simulink model "MPC_Extended_Plant_Simulink"  (R2023b)
settings: Solver=ode4  StartTime=0.0  StopTime=20  FixedStep=1e-3  RelTol=1e-3
values from neighbouring files (symbols this model uses):
  controller_choice = input('Select MPC controller order (1, 2, or 3): ')    [MPC_Extended_Plant.m]    (also in P1.mat = 1; P2.mat = 2; P3.mat = 3)
  init =     [P1.mat]    (also in P2.mat; P3.mat)
  input =     [P1.mat]    (also in P2.mat; P3.mat)
  Np = 40    [MPC_Extended_Plant.m]    (also in P1.mat = 5; P2.mat = 5; P3.mat = 5)
  par =     [P1.mat]    (also in P2.mat; P3.mat)
  Ts = 0.01    [MPC_Extended_Plant.m]    (also in P1.mat; P2.mat; P3.mat)
  V_ref = 16.6666666667    [P1.mat]    (also in P2.mat; P3.mat; veh_parameters.m)
undefined symbols (not defined in the file or in its folder): data
libraries: simulink x12
(part 1 of 2)
settings Model: Creator=bshyrokau  LastModifiedBy=india
settings SolverCC: AlgebraicLoopSolver=TrustRegion
settings DataIOCC: SaveOutput=off  SignalLogging=off  DSMLogging=off  SaveTime=off  ReturnWorkspaceOutputs=off
settings OptimizationCC: ReuseModelBlockBuffer=off  LifeSpan=inf
settings DebuggingCC: UnconnectedInputMsg=warning  UnconnectedOutputMsg=warning  UnconnectedLineMsg=warning  AllowSymbolicDim=off  SFUnexpectedBacktrackingDiag=warning  SFNoUnconditionalDefaultTransitionDiag=warning  SFExecutionAtInitializationDiag=none  ArithmeticOperatorsInVariantConditions=warning
settings ModelReferenceCC: EnableRefExpFcnMdlSchedulingChecks=on  PropagateSignalLabelsOutOfModel=off
settings SFSimCC: SimUseLocalCustomCode=off  CustomCodeUndefinedFunction=UseInterfaceOnly
settings RTWCC: RTWUseLocalCustomCode=off  DLArmComputeVersion=19.05
settings CodeAppCC: StateflowObjectComments=on
settings GRTTargetCC: TargetLangStandard=C89/C90 (ANSI)
settings ConfigComp: CovMetricSettings=dw  CovSaveCumulativeToWorkspaceVar=on  CovSaveSingleToWorkspaceVar=on  CovExternalEMLEnable=off
settings SimscapeCC: SimscapeNormalizeSystem=off
settings ConfigurationSet: Description=SimMechanics 2G

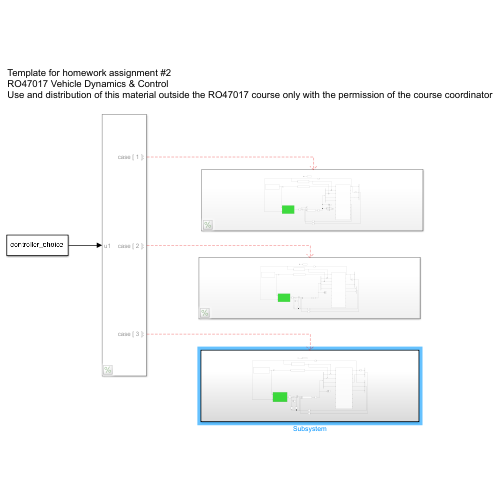
[thumbnail: Simulink's stored preview of the top-level diagram]
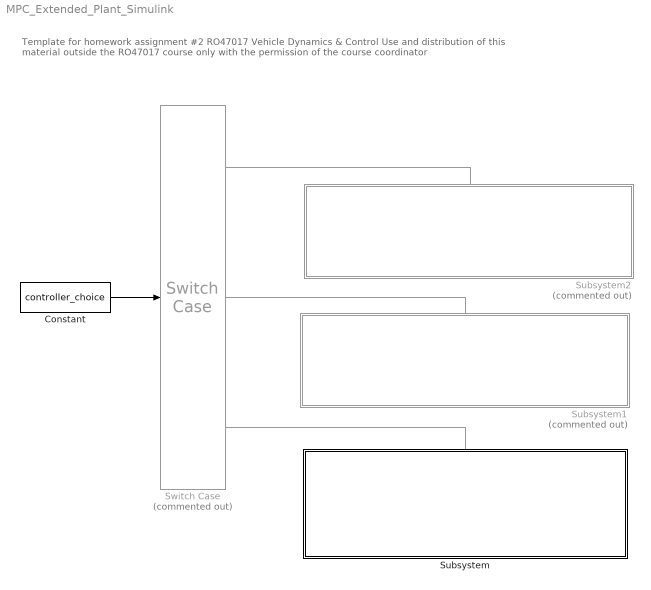
== system MPC_Extended_Plant_Simulink ==
  note: Template for homework assignment #2
      | RO47017 Vehicle Dynamics & Control
      | Use and distribution of this material outside the RO47017 course only with the permission of the course coordinator
  Constant : Constant  Value=controller_choice
  Subsystem : Subsystem
  Subsystem1 : Subsystem  Commented=on
  Subsystem2 : Subsystem  Commented=on
  Switch Case : SwitchCase  Commented=on  CaseConditions={1 2 3}  ShowDefaultCase=off
  wires:
  Switch Case/2 -> ?
  Switch Case/3 -> ?
  Constant/1 -> Switch Case/1
  Switch Case/1 -> ?

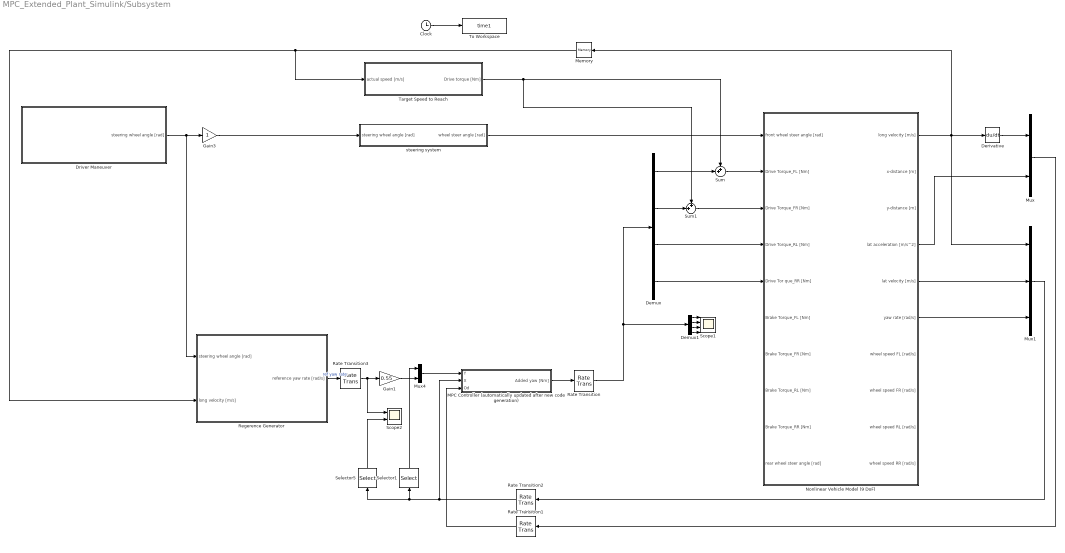
== system MPC_Extended_Plant_Simulink/Subsystem ==
  Clock : Clock
  Demux : Demux
  Demux1 : Demux
  Derivative : Derivative
  Driver Maneuver : Subsystem
  Gain1 : Gain  Gain=0.55
  Gain3 : Gain
  MPC Controller (automatically updated after new code generation) : Subsystem
  Memory : Memory  InitialCondition=V_ref
  Mux : Mux  Inputs=2
  Mux1 : Mux  Inputs=3
  Mux4 : Mux  Inputs=2
  Nonlinear Vehicle Model (9 DoF) : Subsystem
      mask help: Simulink:masks:GenSFuncDesc_MD
      mask Help: eval('feval(''rtwprivate'',''rtwhelpview'',''rtw_sfcn_block'')');
  Rate Transition : RateTransition
  Rate Transition1 : RateTransition  InitialCondition=[0 0]  OutPortSampleTime=Ts
  Rate Transition2 : RateTransition  OutPortSampleTime=Ts
  Rate Transition3 : RateTransition  OutPortSampleTime=Ts
  Regerence Generator : Subsystem
  Scope1 : Scope  NumInputPorts=4
  Scope2 : Scope  NumInputPorts=2
  Selector1 : Selector  InputPortWidth=3  IndexOptions=Index vector (dialog)  Indices=[1 2]  OutputSizes=1
  Selector5 : Selector  InputPortWidth=3  IndexOptions=Index vector (dialog)  Indices=3  OutputSizes=1
  Sum : Sum  Inputs=++|
  Sum1 : Sum  Inputs=++|
  Target Speed to Reach : Subsystem
  To Workspace : ToWorkspace  VariableName=time1  SampleTime=-1
  steering system : Subsystem
  wires:
  Gain1/1 -> Mux4/2
  Selector1/1 -> Mux4/1
  Selector5/1 -> Scope2/2
  Regerence Generator/1(reference yaw rate [rad/s]) -> Rate Transition3/1  "ref yaw rate"
  Target Speed to Reach/1(Drive torque [Nm]) -> Sum/1, Sum1/1
  Demux1/4 -> Scope1/4
  MPC Controller (automatically updated after new code generation)/1(Added yaw [Nm]) -> Rate Transition/1
  Demux/1 -> Sum/2
  Gain3/1 -> steering system/1(steering wheel angle [rad])
  Memory/1 -> Target Speed to Reach/1(actual speed [m/s]), Regerence Generator/2(long velocity [m/s])
  Nonlinear Vehicle Model (9 DoF)/1(long velocity [m/s]) -> Derivative/1, Memory/1, Mux1/1
  Sum/1 -> Nonlinear Vehicle Model (9 DoF)/2(Drive Torque_FL [Nm])
  steering system/1(wheel steer angle [rad]) -> Nonlinear Vehicle Model (9 DoF)/1(front wheel steer angle [rad])
  Rate Transition/1 -> Demux1/1, Demux/1
  Demux1/1 -> Scope1/1
  Demux/3 -> Nonlinear Vehicle Model (9 DoF)/4(Drive Torque_RL [Nm])
  Demux/4 -> Nonlinear Vehicle Model (9 DoF)/5(Drive Tor	que_RR [Nm])
  Demux1/2 -> Scope1/2
  Driver Maneuver/1(steering wheel angle [rad]) -> Gain3/1, Regerence Generator/1(steering wheel angle [rad])
  Mux4/1 -> MPC Controller (automatically updated after new code generation)/1(Y)
  Clock/1 -> To Workspace/1
  Sum1/1 -> Nonlinear Vehicle Model (9 DoF)/3(Drive Torque_FR [Nm])
  Rate Transition2/1 -> Selector5/1, Selector1/1, MPC Controller (automatically updated after new code generation)/2(X)
  Mux1/1 -> Rate Transition2/1
  Demux/2 -> Sum1/2
  Demux1/3 -> Scope1/3
  Rate Transition3/1 -> Scope2/1, Gain1/1
  Nonlinear Vehicle Model (9 DoF)/6(yaw rate [rad/s]) -> Mux1/3
  Nonlinear Vehicle Model (9 DoF)/5(lat velocity [m/s]) -> Mux1/2
  Derivative/1 -> Mux/1
  Nonlinear Vehicle Model (9 DoF)/4(lat acceleration [m/s^2]) -> Mux/2
  Mux/1 -> Rate Transition1/1
  Rate Transition1/1 -> MPC Controller (automatically updated after new code generation)/3(Od)

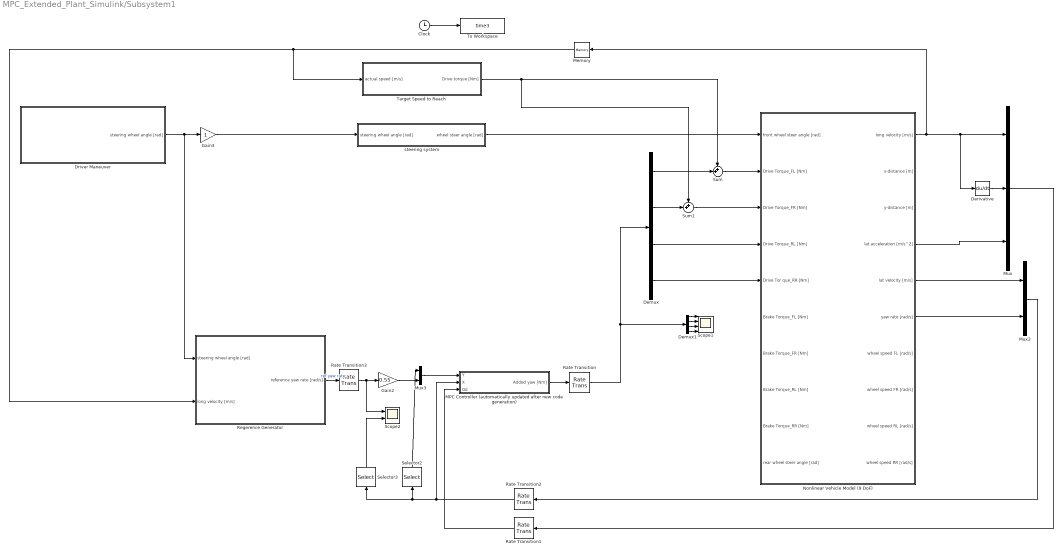
== system MPC_Extended_Plant_Simulink/Subsystem1 ==
  Clock : Clock
  Demux : Demux
  Demux1 : Demux
  Derivative : Derivative
  Driver Maneuver : Subsystem
  Gain2 : Gain  Gain=0.55
  Gain3 : Gain
  MPC Controller (automatically updated after new code generation) : Subsystem
  Memory : Memory  InitialCondition=V_ref
  Mux : Mux  Inputs=3
  Mux2 : Mux  Inputs=2
  Mux3 : Mux  Inputs=2
  Nonlinear Vehicle Model (9 DoF) : Subsystem
      mask help: Simulink:masks:GenSFuncDesc_MD
      mask Help: eval('feval(''rtwprivate'',''rtwhelpview'',''rtw_sfcn_block'')');
  Rate Transition : RateTransition
  Rate Transition1 : RateTransition  InitialCondition=[V_ref 0 0]  OutPortSampleTime=Ts
  Rate Transition2 : RateTransition  OutPortSampleTime=Ts
  Rate Transition3 : RateTransition  OutPortSampleTime=Ts
  Regerence Generator : Subsystem
  Scope1 : Scope  NumInputPorts=4
  Scope2 : Scope  NumInputPorts=2
  Selector2 : Selector  InputPortWidth=2  IndexOptions=Index vector (dialog)  Indices=1  OutputSizes=1
  Selector3 : Selector  InputPortWidth=2  IndexOptions=Index vector (dialog)  Indices=2  OutputSizes=1
  Sum : Sum  Inputs=++|
  Sum1 : Sum  Inputs=++|
  Target Speed to Reach : Subsystem
  To Workspace : ToWorkspace  VariableName=time3  SampleTime=-1
  steering system : Subsystem
  wires:
  Demux1/2 -> Scope1/2
  Demux1/1 -> Scope1/1
  Rate Transition/1 -> Demux1/1, Demux/1
  Demux/3 -> Nonlinear Vehicle Model (9 DoF)/4(Drive Torque_RL [Nm])
  Demux/4 -> Nonlinear Vehicle Model (9 DoF)/5(Drive Tor	que_RR [Nm])
  Sum/1 -> Nonlinear Vehicle Model (9 DoF)/2(Drive Torque_FL [Nm])
  steering system/1(wheel steer angle [rad]) -> Nonlinear Vehicle Model (9 DoF)/1(front wheel steer angle [rad])
  Nonlinear Vehicle Model (9 DoF)/1(long velocity [m/s]) -> Derivative/1, Mux/1, Memory/1
  Demux1/3 -> Scope1/3
  Memory/1 -> Target Speed to Reach/1(actual speed [m/s]), Regerence Generator/2(long velocity [m/s])
  Demux/1 -> Sum/2
  Gain3/1 -> steering system/1(steering wheel angle [rad])
  Demux1/4 -> Scope1/4
  MPC Controller (automatically updated after new code generation)/1(Added yaw [Nm]) -> Rate Transition/1
  Target Speed to Reach/1(Drive torque [Nm]) -> Sum/1, Sum1/1
  Regerence Generator/1(reference yaw rate [rad/s]) -> Rate Transition3/1  "ref yaw rate"
  Demux/2 -> Sum1/2
  Sum1/1 -> Nonlinear Vehicle Model (9 DoF)/3(Drive Torque_FR [Nm])
  Rate Transition3/1 -> Scope2/1, Gain2/1
  Clock/1 -> To Workspace/1
  Rate Transition2/1 -> Selector3/1, Selector2/1, MPC Controller (automatically updated after new code generation)/2(X)
  Driver Maneuver/1(steering wheel angle [rad]) -> Gain3/1, Regerence Generator/1(steering wheel angle [rad])
  Nonlinear Vehicle Model (9 DoF)/5(lat velocity [m/s]) -> Mux2/1
  Nonlinear Vehicle Model (9 DoF)/6(yaw rate [rad/s]) -> Mux2/2
  Mux2/1 -> Rate Transition2/1
  Mux3/1 -> MPC Controller (automatically updated after new code generation)/1(Y)
  Gain2/1 -> Mux3/2
  Selector2/1 -> Mux3/1
  Selector3/1 -> Scope2/2
  Nonlinear Vehicle Model (9 DoF)/4(lat acceleration [m/s^2]) -> Mux/3
  Derivative/1 -> Mux/2
  Mux/1 -> Rate Transition1/1
  Rate Transition1/1 -> MPC Controller (automatically updated after new code generation)/3(Od)

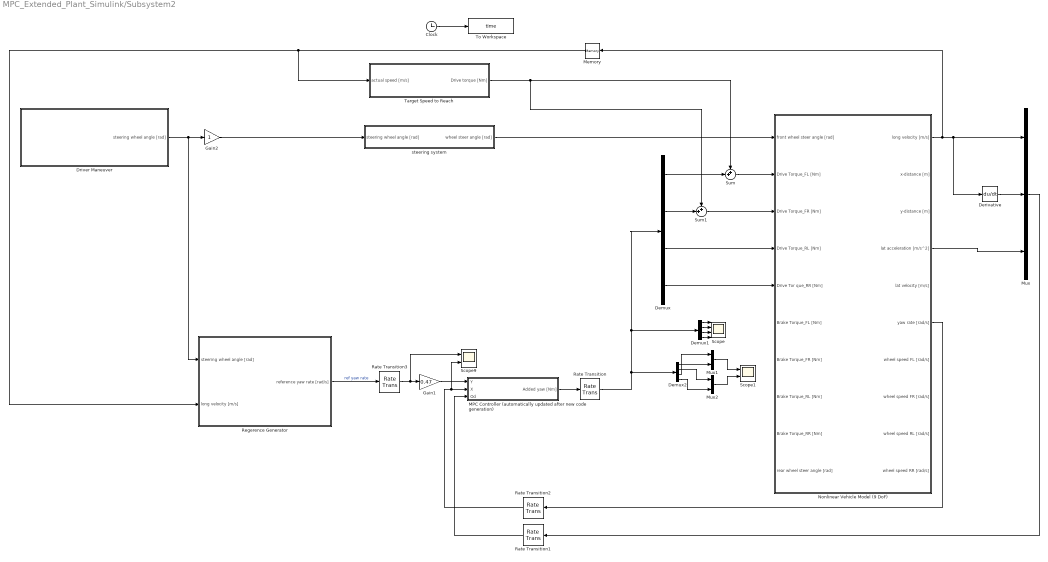
== system MPC_Extended_Plant_Simulink/Subsystem2 ==
  Clock : Clock
  Demux : Demux
  Demux1 : Demux
  Demux2 : Demux
  Derivative : Derivative
  Driver Maneuver : Subsystem
  Gain1 : Gain  Gain=0.47
  Gain2 : Gain
  MPC Controller (automatically updated after new code generation) : Subsystem
  Memory : Memory  InitialCondition=V_ref
  Mux : Mux  Inputs=3
  Mux1 : Mux  Inputs=2
  Mux2 : Mux  Inputs=2
  Nonlinear Vehicle Model (9 DoF) : Subsystem
      mask help: Simulink:masks:GenSFuncDesc_MD
      mask Help: eval('feval(''rtwprivate'',''rtwhelpview'',''rtw_sfcn_block'')');
  Rate Transition : RateTransition  InitialCondition=[0 0 0 0]
  Rate Transition1 : RateTransition  InitialCondition=[V_ref 0 0]  OutPortSampleTime=Ts
  Rate Transition2 : RateTransition  OutPortSampleTime=Ts
  Rate Transition3 : RateTransition  OutPortSampleTime=Ts
  Regerence Generator : Subsystem
  Scope : Scope  NumInputPorts=4
  Scope1 : Scope  NumInputPorts=2
  Scope9 : Scope  NumInputPorts=2
  Sum : Sum  Inputs=++|
  Sum1 : Sum  Inputs=++|
  Target Speed to Reach : Subsystem
  To Workspace : ToWorkspace  VariableName=time  SampleTime=-1
  steering system : Subsystem
  wires:
  MPC Controller (automatically updated after new code generation)/1(Added yaw [Nm]) -> Rate Transition/1
  Gain1/1 -> MPC Controller (automatically updated after new code generation)/1(Y)
  Rate Transition2/1 -> Scope9/2, MPC Controller (automatically updated after new code generation)/2(X)
  Rate Transition3/1 -> Gain1/1, Scope9/1
  Clock/1 -> To Workspace/1
  Regerence Generator/1(reference yaw rate [rad/s]) -> Rate Transition3/1  "ref yaw rate"
  Driver Maneuver/1(steering wheel angle [rad]) -> Gain2/1, Regerence Generator/1(steering wheel angle [rad])
  Gain2/1 -> steering system/1(steering wheel angle [rad])
  steering system/1(wheel steer angle [rad]) -> Nonlinear Vehicle Model (9 DoF)/1(front wheel steer angle [rad])
  Nonlinear Vehicle Model (9 DoF)/6(yaw rate [rad/s]) -> Rate Transition2/1
  Target Speed to Reach/1(Drive torque [Nm]) -> Sum/1, Sum1/1
  Memory/1 -> Target Speed to Reach/1(actual speed [m/s]), Regerence Generator/2(long velocity [m/s])
  Nonlinear Vehicle Model (9 DoF)/1(long velocity [m/s]) -> Memory/1, Derivative/1, Mux/1
  Demux/3 -> Nonlinear Vehicle Model (9 DoF)/4(Drive Torque_RL [Nm])
  Demux/4 -> Nonlinear Vehicle Model (9 DoF)/5(Drive Tor	que_RR [Nm])
  Demux/1 -> Sum/2
  Sum/1 -> Nonlinear Vehicle Model (9 DoF)/2(Drive Torque_FL [Nm])
  Sum1/1 -> Nonlinear Vehicle Model (9 DoF)/3(Drive Torque_FR [Nm])
  Demux/2 -> Sum1/2
  Rate Transition/1 -> Demux2/1, Demux1/1, Demux/1
  Demux1/1 -> Scope/1
  Demux1/2 -> Scope/2
  Demux1/3 -> Scope/3
  Demux1/4 -> Scope/4
  Nonlinear Vehicle Model (9 DoF)/4(lat acceleration [m/s^2]) -> Mux/3
  Derivative/1 -> Mux/2
  Rate Transition1/1 -> MPC Controller (automatically updated after new code generation)/3(Od)
  Mux/1 -> Rate Transition1/1
  Demux2/1 -> Mux1/1
  Demux2/3 -> Mux1/2
  Demux2/2 -> Mux2/1
  Demux2/4 -> Mux2/2
  Mux1/1 -> Scope1/1
  Mux2/1 -> Scope1/2

== system MPC_Extended_Plant_Simulink/Subsystem/Driver Maneuver ==
  Constant1 : Constant
  Lookup Table1 : Lookup  InputValues=[0:0.1:3*pi/2 3*pi/2+eps]*0.7  Table=sin([0:0.1:3*pi/2 3*pi/2+eps])  LookUpMeth=Interpolation-Use End Values  SaturateOnIntegerOverflow=off
  Lookup Table2 : Lookup  InputValues=[3*pi/2:0.1:2*pi 2*pi+eps]*0.7  Table=sin([3*pi/2:0.1:2*pi 2*pi+eps])  LookUpMeth=Interpolation-Use End Values  SaturateOnIntegerOverflow=off
  Ramp2 : simulink/Sources/Ramp  slope=1  start=10  InitialOutput=0
  Ramp6 : simulink/Sources/Ramp  slope=pi  start=10  InitialOutput=0
  Ramp7 : simulink/Sources/Ramp  slope=pi  start=10+0.5  InitialOutput=0
  Sine Wave : Sin  TimeSource=Use external signal  Amplitude=30/180*pi  Frequency=2*pi*0.2  SampleTime=0
  Subtract1 : Sum  Inputs=+++
  Terminator1 : Terminator
  amplitude : Gain  Gain=120
  deg2rad : Gain  Gain=pi / 180
  steering wheel angle [rad] : Outport  VectorParamsAs1DForOutWhenUnconnected=off
  wires:
  Ramp6/1 -> Lookup Table1/1
  Ramp7/1 -> Lookup Table2/1
  Lookup Table2/1 -> Subtract1/2
  Lookup Table1/1 -> Subtract1/1
  Constant1/1 -> Subtract1/3
  Subtract1/1 -> amplitude/1
  amplitude/1 -> deg2rad/1
  Ramp2/1 -> Sine Wave/1
  deg2rad/1 -> steering wheel angle [rad]/1
  Sine Wave/1 -> Terminator1/1

== system MPC_Extended_Plant_Simulink/Subsystem/MPC Controller (automatically updated after new code generation) ==
  Y : Inport
  X : Inport  Port=2
  Od : Inport  Port=3
  Bus Assignment : BusAssignment  AssignedSignals=data.x0,data.y,data.yN,data.W,data.WN,data.od
  Bus Creator : BusCreator  Inputs=4  OutDataTypeStr=Bus: ACADOinput
  Bus Selector : BusSelector  OutputSignals=data
  Bus Selector1 : BusSelector  OutputSignals=data.u
  Initial conditions : Constant  Value=[V_ref 0 0]
  Selector : Selector  InputPortWidth=Np*4  IndexOptions=Starting index (dialog)  Indices=1  OutputSizes=4
  Shift reference : MATLAB Function  TreatAsAtomicUnit=on
  Shift reference1 : MATLAB Function  TreatAsAtomicUnit=on
  Unit Delay : UnitDelay  InitialCondition=init  SampleTime=Ts  HasFrameUpgradeWarning=on
  acado_solver_sfun : S-Function  FunctionName=acado_solver_sfun  SFunctionDeploymentMode=off  EnableBusSupport=off  mask(Legacy Function){SFunctionSpec=acado_step(ACADOinput u1[1], ACADOoutput y1[1]), ShowSpec=on}
      mask prompts: ShowSpec "Display function specification"
      mask help:
      | This block allows you to call the legacy functions specified by the following Legacy Code Tool definition:
      | def.SFunctionName = 'acado_solver_sfun';
      | def.OutputFcnSpec = 'acado_step(ACADOinput u1[1], ACADOoutput y1[1])';
      | def.StartFcnSpec = 'acado_initialize( void )';
      | def.TerminateFcnSpec = 'acado_cleanup( void )';
      | def.HeaderFiles = {'acado_common.h', 'acado_solver_sfunction.h'};
      | def.SourceFiles = {'acado_solver.c', 'acado_integrator.c', 'acado_auxiliary_functions.c', 'acado_solver_sfunction.c', 'acado_qpoases3_interface.c', 'qpoases3\src\Bounds.c', 'qpoases3\src\Constraints.c', 'qpoases3\src\Indexlist.c', 'qpoases3\src\Matrices.c', 'qpoases3\src\MessageHandling.c', 'qpoases3\src\Options.c', 'qpoases3\src\Flipper.c', 'qpoases3\src\QProblem.c', 'qpoases3\src\QProblemB.c', 'qpoases3\src\Utils.c'};
      mask Help: <p>This block was generated automatically by the Legacy Code Tool. For detailed help on this tool, call<a href="matlab:legacy_code('help')"> legacy_code('help')</a>.</p>
      mask Callback ShowSpec:
      | if strcmp(get_param(gcbh, 'ShowSpec'), 'on')
      |   set_param(gcbh, 'MaskDisplay', sprintf('fprintf(''%s'');', get_param(gcbh, 'SFunctionSpec')));
      | else
      |   set_param(gcbh, 'MaskDisplay', sprintf('fprintf(''%s'');', get_param(gcbh, 'FunctionName')));
      | end
      mask Display: fprintf('acado_step(ACADOinput u1[1], ACADOoutput y1[1])');
  control : Constant  Value=0  OutDataTypeStr=int32
  initialization : Constant  Value=0  OutDataTypeStr=int32
  shifting : Constant  OutDataTypeStr=int32
  stage cost matrix : Constant  Value=reshape(diag([0 0 7e8 1 1 1 1]),1,length(input.W)^2)
  terminal cost matrix : Constant  Value=reshape(diag([0 0 0]),1,length(input.WN)^2)
  Added yaw [Nm] : Outport
  wires:
  control/1 -> Bus Creator/1  "control"
  Bus Selector1/1 -> Selector/1  "<u>"
  initialization/1 -> Bus Creator/3  "initialization"
  acado_solver_sfun/1 -> Bus Selector1/1, Bus Assignment/1
  shifting/1 -> Bus Creator/2  "shifting"
  Bus Assignment/1 -> Bus Selector/1
  terminal cost matrix/1 -> Bus Assignment/6
  Initial conditions/1 -> Bus Assignment/4
  Shift reference/1(y) -> Bus Assignment/3
  stage cost matrix/1 -> Bus Assignment/5
  Bus Selector/1 -> Unit Delay/1  "<data>"
  Unit Delay/1 -> Bus Creator/4
  Bus Creator/1 -> acado_solver_sfun/1
  Selector/1 -> Added yaw [Nm]/1  "delta"
  Y/1 -> Shift reference/1(yN)
  X/1 -> Bus Assignment/2
  Shift reference1/1(y) -> Bus Assignment/7
  Od/1 -> Shift reference1/1(yN)

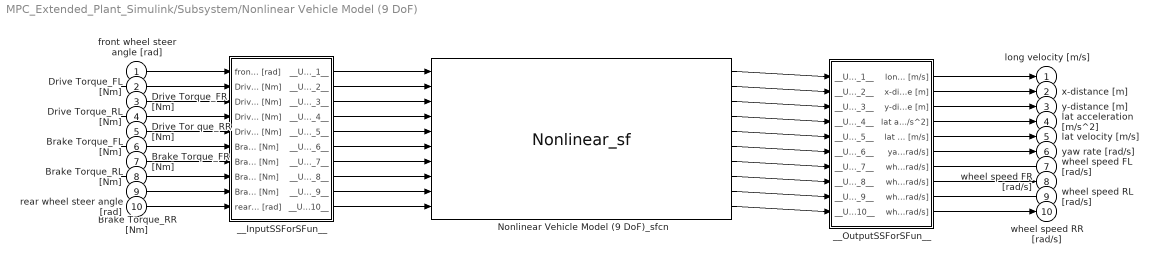
== system MPC_Extended_Plant_Simulink/Subsystem/Nonlinear Vehicle Model (9 DoF) ==
  front wheel steer angle [rad] : Inport
  Drive Torque_FL [Nm] : Inport  Port=2
  Drive Torque_FR [Nm] : Inport  Port=3
  Drive Torque_RL [Nm] : Inport  Port=4
  Drive Tor	que_RR [Nm] : Inport  Port=5
  Brake Torque_FL [Nm] : Inport  Port=6
  Brake Torque_FR [Nm] : Inport  Port=7
  Brake Torque_RL [Nm] : Inport  Port=8
  Brake Torque_RR [Nm] : Inport  Port=9
  rear wheel steer angle [rad] : Inport  Port=10
  Nonlinear Vehicle Model (9 DoF)_sfcn : S-Function  FunctionName=Nonlinear_sf  SFunctionModules=""  SFunctionDeploymentMode=off  EnableBusSupport=off  mask{rtw_sf_name=Nonlinear_sf, showVar=off}
      mask prompts: rtw_sf_name "Simulink:masks:GenSFuncName_MP"; showVar "Simulink:masks:GenSFuncShowModuleList_MP"
      mask help: Simulink:masks:GenSFuncDesc_MD
      mask init:
      | displist = '';
      | if ~strcmp(get_param(gcb, 'FunctionName'), rtw_sf_name);
      |   set_param(gcb, 'FunctionName', rtw_sf_name);
      | end
      | % Check if we are generating code
      | rtw_mode = false;
      | if strcmpi(get_param(bdroot(gcb),'SimulationStatus'),'Initializing')
      | 	rtw_mode = strcmpi(get_param(bdroot(gcb),'BuildingRTWCode'),'on') && ...
      | 		~strcmpi(get_param(bdroot(gcb),'TargetStyle'),'SimulationTarget');
      | end
      | if showVar || rtw_mode
      | 	if exist('rtwsfunc') == 2 | exist('rtwsfunc') == 6
      | 		tmplist = rtwsfunc(rtw_sf_name,gcb);
      | 		tmplist = DAStudio.message('Simulink:masks:GenSFuncListOfModules_IC', tmplist);
      | 	elseif showVar
      | 		tmplist1 = DAStudio.message('Simulink:masks:GenSFuncListOfModules_IC', '');
      |         tmplist2 = DAStudio.message('Simulink:masks:GenSFuncNotLicensed_IC');
      |         tmplist = [tmplist1 tmplist2];
      |  	end
      | end
      | if showVar
      |   displist = tmplist;
      | end
      settings: CopyFcn=|
      | if ~strcmp(get_param(gcb,'Linkstatus'),'none') && ...
      | ~strcmp(get_param(gcb,'Linkstatus'),'implicit')
      |   set_param(gcb,'LinkStatus','none');
      | end
      mask Help: eval('feval(''rtwprivate'',''rtwhelpview'',''rtw_sfcn_block'')');
      mask Display:
      | port_label('input',1,'front wheel steer angle [rad]');
      | port_label('input',2,'Drive Torque_FL [Nm]');
      | port_label('input',3,'Drive Torque_FR [Nm]');
      | port_label('input',4,'Drive Torque_RL [Nm]');
      | port_label('input',5,'Drive Tor	que_RR [Nm]');
      | port_label('input',6,'Brake Torque_FL [Nm]');
      | port_label('input',7,'Brake Torque_FR [Nm]');
      | port_label('input',8,'Brake Torque_RL [Nm]');
      | port_label('input',9,'Brake Torque_RR [Nm]');
      | port_label('input',10,'rear wheel steer angle [rad]');
      | port_label('output',1,'long velocity [m/s]');
      | port_label('output',2,'x-distance [m]');
      | port_label('output',3,'y-distance [m]');
      | port_label('output',4,'lat acceleration [m/s^2]');
      | port_label('output',5,'lat velocity [m/s]');
      | port_label('output',6,'yaw rate [rad/s]');
      | port_label('output',7,'wheel speed FL [rad/s]');
      | port_label('output',8,'wheel speed FR [rad/s]');
      | port_label('output',9,'wheel speed RL [rad/s]');
      | port_label('output',10,'wheel speed RR [rad/s]');
  __InputSSForSFun__ : Subsystem
  __OutputSSForSFun__ : Subsystem
  long velocity [m/s] : Outport  VectorParamsAs1DForOutWhenUnconnected=off
  x-distance [m] : Outport  Port=2  VectorParamsAs1DForOutWhenUnconnected=off
  y-distance [m] : Outport  Port=3  VectorParamsAs1DForOutWhenUnconnected=off
  lat acceleration [m/s^2] : Outport  Port=4  VectorParamsAs1DForOutWhenUnconnected=off
  lat velocity [m/s] : Outport  Port=5  VectorParamsAs1DForOutWhenUnconnected=off
  yaw rate [rad/s] : Outport  Port=6  VectorParamsAs1DForOutWhenUnconnected=off
  wheel speed FL [rad/s] : Outport  Port=7  VectorParamsAs1DForOutWhenUnconnected=off
  wheel speed FR [rad/s] : Outport  Port=8  VectorParamsAs1DForOutWhenUnconnected=off
  wheel speed RL [rad/s] : Outport  Port=9  VectorParamsAs1DForOutWhenUnconnected=off
  wheel speed RR [rad/s] : Outport  Port=10  VectorParamsAs1DForOutWhenUnconnected=off
  wires:
  front wheel steer angle [rad]/1 -> __InputSSForSFun__/1(front wheel steer angle [rad])
  Drive Torque_FL [Nm]/1 -> __InputSSForSFun__/2(Drive Torque_FL [Nm])
  Drive Torque_FR [Nm]/1 -> __InputSSForSFun__/3(Drive Torque_FR [Nm])
  Drive Torque_RL [Nm]/1 -> __InputSSForSFun__/4(Drive Torque_RL [Nm])
  Drive Tor	que_RR [Nm]/1 -> __InputSSForSFun__/5(Drive Tor	que_RR [Nm])
  Brake Torque_FL [Nm]/1 -> __InputSSForSFun__/6(Brake Torque_FL [Nm])
  Brake Torque_FR [Nm]/1 -> __InputSSForSFun__/7(Brake Torque_FR [Nm])
  Brake Torque_RL [Nm]/1 -> __InputSSForSFun__/8(Brake Torque_RL [Nm])
  Brake Torque_RR [Nm]/1 -> __InputSSForSFun__/9(Brake Torque_RR [Nm])
  rear wheel steer angle [rad]/1 -> __InputSSForSFun__/10(rear wheel steer angle [rad])
  __InputSSForSFun__/1(__UniqueOutportName__1__) -> Nonlinear Vehicle Model (9 DoF)_sfcn/1
  __InputSSForSFun__/2(__UniqueOutportName__2__) -> Nonlinear Vehicle Model (9 DoF)_sfcn/2
  __InputSSForSFun__/3(__UniqueOutportName__3__) -> Nonlinear Vehicle Model (9 DoF)_sfcn/3
  __InputSSForSFun__/4(__UniqueOutportName__4__) -> Nonlinear Vehicle Model (9 DoF)_sfcn/4
  __InputSSForSFun__/5(__UniqueOutportName__5__) -> Nonlinear Vehicle Model (9 DoF)_sfcn/5
  __InputSSForSFun__/6(__UniqueOutportName__6__) -> Nonlinear Vehicle Model (9 DoF)_sfcn/6
  __InputSSForSFun__/7(__UniqueOutportName__7__) -> Nonlinear Vehicle Model (9 DoF)_sfcn/7
  __InputSSForSFun__/8(__UniqueOutportName__8__) -> Nonlinear Vehicle Model (9 DoF)_sfcn/8
  __InputSSForSFun__/9(__UniqueOutportName__9__) -> Nonlinear Vehicle Model (9 DoF)_sfcn/9
  __InputSSForSFun__/10(__UniqueOutportName__10__) -> Nonlinear Vehicle Model (9 DoF)_sfcn/10
  Nonlinear Vehicle Model (9 DoF)_sfcn/1 -> __OutputSSForSFun__/1(__UniqueInportName__1__)
  Nonlinear Vehicle Model (9 DoF)_sfcn/2 -> __OutputSSForSFun__/2(__UniqueInportName__2__)
  Nonlinear Vehicle Model (9 DoF)_sfcn/3 -> __OutputSSForSFun__/3(__UniqueInportName__3__)
  Nonlinear Vehicle Model (9 DoF)_sfcn/4 -> __OutputSSForSFun__/4(__UniqueInportName__4__)
  Nonlinear Vehicle Model (9 DoF)_sfcn/5 -> __OutputSSForSFun__/5(__UniqueInportName__5__)
  Nonlinear Vehicle Model (9 DoF)_sfcn/6 -> __OutputSSForSFun__/6(__UniqueInportName__6__)
  Nonlinear Vehicle Model (9 DoF)_sfcn/7 -> __OutputSSForSFun__/7(__UniqueInportName__7__)
  Nonlinear Vehicle Model (9 DoF)_sfcn/8 -> __OutputSSForSFun__/8(__UniqueInportName__8__)
  Nonlinear Vehicle Model (9 DoF)_sfcn/9 -> __OutputSSForSFun__/9(__UniqueInportName__9__)
  Nonlinear Vehicle Model (9 DoF)_sfcn/10 -> __OutputSSForSFun__/10(__UniqueInportName__10__)
  __OutputSSForSFun__/1(long velocity [m/s]) -> long velocity [m/s]/1
  __OutputSSForSFun__/2(x-distance [m]) -> x-distance [m]/1
  __OutputSSForSFun__/3(y-distance [m]) -> y-distance [m]/1
  __OutputSSForSFun__/4(lat acceleration [m/s^2]) -> lat acceleration [m/s^2]/1
  __OutputSSForSFun__/5(lat velocity [m/s]) -> lat velocity [m/s]/1
  __OutputSSForSFun__/6(yaw rate [rad/s]) -> yaw rate [rad/s]/1
  __OutputSSForSFun__/7(wheel speed FL [rad/s]) -> wheel speed FL [rad/s]/1
  __OutputSSForSFun__/8(wheel speed FR [rad/s]) -> wheel speed FR [rad/s]/1
  __OutputSSForSFun__/9(wheel speed RL [rad/s]) -> wheel speed RL [rad/s]/1
  __OutputSSForSFun__/10(wheel speed RR [rad/s]) -> wheel speed RR [rad/s]/1

== system MPC_Extended_Plant_Simulink/Subsystem/Regerence Generator ==
  note: yawr_ref
  note: nonlinear response
  note: delta
  note: u
  steering wheel angle [rad] : Inport
  long velocity [m/s] : Inport  Port=2
  MATLAB Function : MATLAB Function  TreatAsAtomicUnit=on
  MATLAB Function1 : MATLAB Function  TreatAsAtomicUnit=on
  Transfer Fcn : TransferFcn  Numerator=[par.wn^2*par.tau par.wn^2]  Denominator=[1 2*par.kseta*par.wn par.wn^2]
  steering ratio : Gain  Gain=1/ par.i_steer
  reference yaw rate [rad/s] : Outport  VectorParamsAs1DForOutWhenUnconnected=off
  wires:
  steering wheel angle [rad]/1 -> steering ratio/1
  steering ratio/1 -> MATLAB Function/1(delta)
  long velocity [m/s]/1 -> MATLAB Function1/2(u), MATLAB Function/2(u)
  MATLAB Function/1(yawr_ss) -> MATLAB Function1/1(yawr_ss)
  MATLAB Function1/1(yawr_sat) -> Transfer Fcn/1
  Transfer Fcn/1 -> reference yaw rate [rad/s]/1

== system MPC_Extended_Plant_Simulink/Subsystem/Target Speed to Reach ==
  actual speed [m/s] : Inport
  " " : Lookup_n-D  NumberOfTableDimensions=1  BreakpointsForDimension1="[-10  0  10 30]"  IndexSearchMethod=Linear search  Table=[0.1 0.1 1 1]  ExtrapMethod=Clip  RemoveProtectionInput=on  UseLastTableValue=on  RndMeth=Simplest
  Add : Sum  Inputs=+-
  Add1 : Sum
  Gain : Gain  Gain=1000
  Gain1 : Gain  Gain=10
  Ground3 : Ground
  Integrator1 : Integrator  LimitOutput=on  UpperSaturationLimit=0.1  LowerSaturationLimit=-0.1
  Product : Product  RndMeth=Zero
  Product1 : Product  RndMeth=Zero
  Ramp6 : simulink/Sources/Ramp  slope=1  start=0  InitialOutput=0
  Saturation : Saturate  UpperLimit=1  LowerLimit=0
  Switch : Switch  Criteria=u2 > Threshold  Threshold=8  SaturateOnIntegerOverflow=off  InputSameDT=off
  low-pass (1 Hz) : TransferFcn  Denominator=[1/(2*pi) 1]
  "target pre-maneuver speed [m/s] " : Constant  Value=V_ref
  Drive torque [Nm] : Outport
  wires:
  actual speed [m/s]/1 -> low-pass (1 Hz)/1, Add/2
  "target pre-maneuver speed [m/s] "/1 -> Add/1
  Gain1/1 -> Integrator1/1
  Product/1 -> Add1/1
  Add/1 -> Product/1, Product1/1
  Product1/1 -> Gain1/1
  " "/1 -> Product1/2, Product/2
  low-pass (1 Hz)/1 -> " "/1
  Add1/1 -> Saturation/1
  Integrator1/1 -> Add1/2
  Ramp6/1 -> Switch/2
  Switch/1 -> Gain/1
  Ground3/1 -> Switch/1
  Saturation/1 -> Switch/3
  Gain/1 -> Drive torque [Nm]/1

== system MPC_Extended_Plant_Simulink/Subsystem/steering system ==
  steering wheel angle [rad] : Inport
  Delay : TransportDelay  DelayTime=par.teta_ss
  Steering Dynamics : TransferFcn  Numerator=[par.wn_ss^2]  Denominator=[1 2*par.zeta_ss*par.wn_ss par.wn_ss^2]
  steering ratio : Gain  Gain=1/ par.i_steer
  wheel steer angle [rad] : Outport  VectorParamsAs1DForOutWhenUnconnected=off
  wires:
  steering wheel angle [rad]/1 -> steering ratio/1
  Delay/1 -> Steering Dynamics/1
  steering ratio/1 -> Delay/1
  Steering Dynamics/1 -> wheel steer angle [rad]/1

== system MPC_Extended_Plant_Simulink/Subsystem1/Driver Maneuver ==
  Constant1 : Constant
  Lookup Table1 : Lookup  InputValues=[0:0.1:3*pi/2 3*pi/2+eps]*0.7  Table=sin([0:0.1:3*pi/2 3*pi/2+eps])  LookUpMeth=Interpolation-Use End Values  SaturateOnIntegerOverflow=off
  Lookup Table2 : Lookup  InputValues=[3*pi/2:0.1:2*pi 2*pi+eps]*0.7  Table=sin([3*pi/2:0.1:2*pi 2*pi+eps])  LookUpMeth=Interpolation-Use End Values  SaturateOnIntegerOverflow=off
  Ramp2 : simulink/Sources/Ramp  slope=1  start=10  InitialOutput=0
  Ramp6 : simulink/Sources/Ramp  slope=pi  start=10  InitialOutput=0
  Ramp7 : simulink/Sources/Ramp  slope=pi  start=10+0.5  InitialOutput=0
  Sine Wave : Sin  TimeSource=Use external signal  Amplitude=30/180*pi  Frequency=2*pi*0.2  SampleTime=0
  Subtract1 : Sum  Inputs=+++
  Terminator1 : Terminator
  amplitude : Gain  Gain=120
  deg2rad : Gain  Gain=pi / 180
  steering wheel angle [rad] : Outport  VectorParamsAs1DForOutWhenUnconnected=off
  wires:
  Ramp6/1 -> Lookup Table1/1
  Ramp7/1 -> Lookup Table2/1
  Lookup Table2/1 -> Subtract1/2
  Lookup Table1/1 -> Subtract1/1
  Constant1/1 -> Subtract1/3
  Subtract1/1 -> amplitude/1
  amplitude/1 -> deg2rad/1
  Ramp2/1 -> Sine Wave/1
  deg2rad/1 -> steering wheel angle [rad]/1
  Sine Wave/1 -> Terminator1/1

== system MPC_Extended_Plant_Simulink/Subsystem1/MPC Controller (automatically updated after new code generation) ==
  Y : Inport
  X : Inport  Port=2
  Od : Inport  Port=3
  Bus Assignment : BusAssignment  AssignedSignals=data.x0,data.y,data.yN,data.W,data.WN,data.od
  Bus Creator : BusCreator  Inputs=4  OutDataTypeStr=Bus: ACADOinput
  Bus Selector : BusSelector  OutputSignals=data
  Bus Selector1 : BusSelector  OutputSignals=data.u
  Initial conditions : Constant  Value=[0 0]
  Selector : Selector  InputPortWidth=Np*4  IndexOptions=Starting index (dialog)  Indices=1  OutputSizes=4
  Shift reference : MATLAB Function  TreatAsAtomicUnit=on
  Shift reference2 : MATLAB Function  TreatAsAtomicUnit=on
  Unit Delay : UnitDelay  InitialCondition=init  SampleTime=Ts  HasFrameUpgradeWarning=on
  acado_solver_sfun : S-Function  FunctionName=acado_solver_sfun  SFunctionDeploymentMode=off  EnableBusSupport=off  mask(Legacy Function){SFunctionSpec=acado_step(ACADOinput u1[1], ACADOoutput y1[1]), ShowSpec=on}
      mask prompts: ShowSpec "Display function specification"
      mask help:
      | This block allows you to call the legacy functions specified by the following Legacy Code Tool definition:
      | def.SFunctionName = 'acado_solver_sfun';
      | def.OutputFcnSpec = 'acado_step(ACADOinput u1[1], ACADOoutput y1[1])';
      | def.StartFcnSpec = 'acado_initialize( void )';
      | def.TerminateFcnSpec = 'acado_cleanup( void )';
      | def.HeaderFiles = {'acado_common.h', 'acado_solver_sfunction.h'};
      | def.SourceFiles = {'acado_solver.c', 'acado_integrator.c', 'acado_auxiliary_functions.c', 'acado_solver_sfunction.c', 'acado_qpoases3_interface.c', 'qpoases3\src\Bounds.c', 'qpoases3\src\Constraints.c', 'qpoases3\src\Indexlist.c', 'qpoases3\src\Matrices.c', 'qpoases3\src\MessageHandling.c', 'qpoases3\src\Options.c', 'qpoases3\src\Flipper.c', 'qpoases3\src\QProblem.c', 'qpoases3\src\QProblemB.c', 'qpoases3\src\Utils.c'};
      mask Help: <p>This block was generated automatically by the Legacy Code Tool. For detailed help on this tool, call<a href="matlab:legacy_code('help')"> legacy_code('help')</a>.</p>
      mask Callback ShowSpec:
      | if strcmp(get_param(gcbh, 'ShowSpec'), 'on')
      |   set_param(gcbh, 'MaskDisplay', sprintf('fprintf(''%s'');', get_param(gcbh, 'SFunctionSpec')));
      | else
      |   set_param(gcbh, 'MaskDisplay', sprintf('fprintf(''%s'');', get_param(gcbh, 'FunctionName')));
      | end
      mask Display: fprintf('acado_step(ACADOinput u1[1], ACADOoutput y1[1])');
  control : Constant  Value=0  OutDataTypeStr=int32
  initialization : Constant  Value=0  OutDataTypeStr=int32
  shifting : Constant  OutDataTypeStr=int32
  stage cost matrix : Constant  Value=reshape(diag([0 7e8 1 1 1 1]),1,length(input.W)^2)
  terminal cost matrix : Constant  Value=reshape(diag([0 0]),1,length(input.WN)^2)
  Added yaw [Nm] : Outport
  wires:
  control/1 -> Bus Creator/1  "control"
  Bus Selector1/1 -> Selector/1  "<u>"
  initialization/1 -> Bus Creator/3  "initialization"
  acado_solver_sfun/1 -> Bus Selector1/1, Bus Assignment/1
  shifting/1 -> Bus Creator/2  "shifting"
  Bus Assignment/1 -> Bus Selector/1
  terminal cost matrix/1 -> Bus Assignment/6
  Initial conditions/1 -> Bus Assignment/4
  Shift reference/1(y) -> Bus Assignment/3
  stage cost matrix/1 -> Bus Assignment/5
  Bus Selector/1 -> Unit Delay/1  "<data>"
  Unit Delay/1 -> Bus Creator/4
  Bus Creator/1 -> acado_solver_sfun/1
  Selector/1 -> Added yaw [Nm]/1  "delta"
  Y/1 -> Shift reference/1(yN)
  X/1 -> Bus Assignment/2
  Shift reference2/1(y) -> Bus Assignment/7
  Od/1 -> Shift reference2/1(yN)

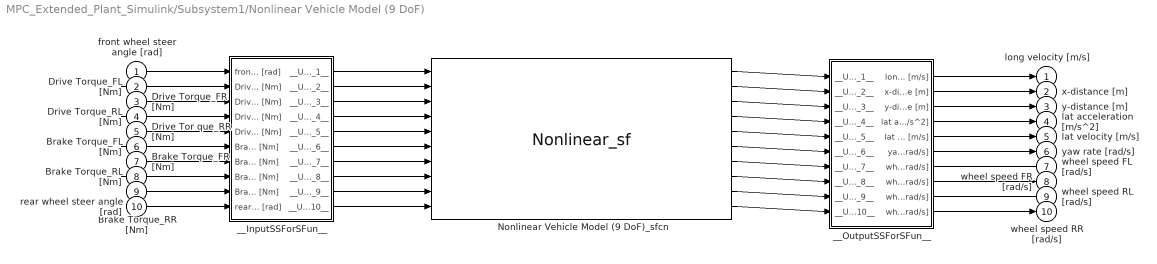
== system MPC_Extended_Plant_Simulink/Subsystem1/Nonlinear Vehicle Model (9 DoF) ==
  front wheel steer angle [rad] : Inport
  Drive Torque_FL [Nm] : Inport  Port=2
  Drive Torque_FR [Nm] : Inport  Port=3
  Drive Torque_RL [Nm] : Inport  Port=4
  Drive Tor	que_RR [Nm] : Inport  Port=5
  Brake Torque_FL [Nm] : Inport  Port=6
  Brake Torque_FR [Nm] : Inport  Port=7
  Brake Torque_RL [Nm] : Inport  Port=8
  Brake Torque_RR [Nm] : Inport  Port=9
  rear wheel steer angle [rad] : Inport  Port=10
  Nonlinear Vehicle Model (9 DoF)_sfcn : S-Function  FunctionName=Nonlinear_sf  SFunctionModules=""  SFunctionDeploymentMode=off  EnableBusSupport=off  mask{rtw_sf_name=Nonlinear_sf, showVar=off}
      mask prompts: rtw_sf_name "Simulink:masks:GenSFuncName_MP"; showVar "Simulink:masks:GenSFuncShowModuleList_MP"
      mask help: Simulink:masks:GenSFuncDesc_MD
      mask init: same as MPC_Extended_Plant_Simulink/Subsystem/Nonlinear Vehicle Model (9 DoF)/Nonlinear Vehicle Model (9 DoF)_sfcn
      settings: CopyFcn=|
      | if ~strcmp(get_param(gcb,'Linkstatus'),'none') && ...
      | ~strcmp(get_param(gcb,'Linkstatus'),'implicit')
      |   set_param(gcb,'LinkStatus','none');
      | end
      mask Help: eval('feval(''rtwprivate'',''rtwhelpview'',''rtw_sfcn_block'')');
      mask Display:
      | port_label('input',1,'front wheel steer angle [rad]');
      | port_label('input',2,'Drive Torque_FL [Nm]');
      | port_label('input',3,'Drive Torque_FR [Nm]');
      | port_label('input',4,'Drive Torque_RL [Nm]');
      | port_label('input',5,'Drive Tor	que_RR [Nm]');
      | port_label('input',6,'Brake Torque_FL [Nm]');
      | port_label('input',7,'Brake Torque_FR [Nm]');
      | port_label('input',8,'Brake Torque_RL [Nm]');
      | port_label('input',9,'Brake Torque_RR [Nm]');
      | port_label('input',10,'rear wheel steer angle [rad]');
      | port_label('output',1,'long velocity [m/s]');
      | port_label('output',2,'x-distance [m]');
      | port_label('output',3,'y-distance [m]');
      | port_label('output',4,'lat acceleration [m/s^2]');
      | port_label('output',5,'lat velocity [m/s]');
      | port_label('output',6,'yaw rate [rad/s]');
      | port_label('output',7,'wheel speed FL [rad/s]');
      | port_label('output',8,'wheel speed FR [rad/s]');
      | port_label('output',9,'wheel speed RL [rad/s]');
      | port_label('output',10,'wheel speed RR [rad/s]');
  __InputSSForSFun__ : Subsystem
  __OutputSSForSFun__ : Subsystem
  long velocity [m/s] : Outport  VectorParamsAs1DForOutWhenUnconnected=off
  x-distance [m] : Outport  Port=2  VectorParamsAs1DForOutWhenUnconnected=off
  y-distance [m] : Outport  Port=3  VectorParamsAs1DForOutWhenUnconnected=off
  lat acceleration [m/s^2] : Outport  Port=4  VectorParamsAs1DForOutWhenUnconnected=off
  lat velocity [m/s] : Outport  Port=5  VectorParamsAs1DForOutWhenUnconnected=off
  yaw rate [rad/s] : Outport  Port=6  VectorParamsAs1DForOutWhenUnconnected=off
  wheel speed FL [rad/s] : Outport  Port=7  VectorParamsAs1DForOutWhenUnconnected=off
  wheel speed FR [rad/s] : Outport  Port=8  VectorParamsAs1DForOutWhenUnconnected=off
  wheel speed RL [rad/s] : Outport  Port=9  VectorParamsAs1DForOutWhenUnconnected=off
  wheel speed RR [rad/s] : Outport  Port=10  VectorParamsAs1DForOutWhenUnconnected=off
  wires:
  front wheel steer angle [rad]/1 -> __InputSSForSFun__/1(front wheel steer angle [rad])
  Drive Torque_FL [Nm]/1 -> __InputSSForSFun__/2(Drive Torque_FL [Nm])
  Drive Torque_FR [Nm]/1 -> __InputSSForSFun__/3(Drive Torque_FR [Nm])
  Drive Torque_RL [Nm]/1 -> __InputSSForSFun__/4(Drive Torque_RL [Nm])
  Drive Tor	que_RR [Nm]/1 -> __InputSSForSFun__/5(Drive Tor	que_RR [Nm])
  Brake Torque_FL [Nm]/1 -> __InputSSForSFun__/6(Brake Torque_FL [Nm])
  Brake Torque_FR [Nm]/1 -> __InputSSForSFun__/7(Brake Torque_FR [Nm])
  Brake Torque_RL [Nm]/1 -> __InputSSForSFun__/8(Brake Torque_RL [Nm])
  Brake Torque_RR [Nm]/1 -> __InputSSForSFun__/9(Brake Torque_RR [Nm])
  rear wheel steer angle [rad]/1 -> __InputSSForSFun__/10(rear wheel steer angle [rad])
  __InputSSForSFun__/1(__UniqueOutportName__1__) -> Nonlinear Vehicle Model (9 DoF)_sfcn/1
  __InputSSForSFun__/2(__UniqueOutportName__2__) -> Nonlinear Vehicle Model (9 DoF)_sfcn/2
  __InputSSForSFun__/3(__UniqueOutportName__3__) -> Nonlinear Vehicle Model (9 DoF)_sfcn/3
  __InputSSForSFun__/4(__UniqueOutportName__4__) -> Nonlinear Vehicle Model (9 DoF)_sfcn/4
  __InputSSForSFun__/5(__UniqueOutportName__5__) -> Nonlinear Vehicle Model (9 DoF)_sfcn/5
  __InputSSForSFun__/6(__UniqueOutportName__6__) -> Nonlinear Vehicle Model (9 DoF)_sfcn/6
  __InputSSForSFun__/7(__UniqueOutportName__7__) -> Nonlinear Vehicle Model (9 DoF)_sfcn/7
  __InputSSForSFun__/8(__UniqueOutportName__8__) -> Nonlinear Vehicle Model (9 DoF)_sfcn/8
  __InputSSForSFun__/9(__UniqueOutportName__9__) -> Nonlinear Vehicle Model (9 DoF)_sfcn/9
  __InputSSForSFun__/10(__UniqueOutportName__10__) -> Nonlinear Vehicle Model (9 DoF)_sfcn/10
  Nonlinear Vehicle Model (9 DoF)_sfcn/1 -> __OutputSSForSFun__/1(__UniqueInportName__1__)
  Nonlinear Vehicle Model (9 DoF)_sfcn/2 -> __OutputSSForSFun__/2(__UniqueInportName__2__)
  Nonlinear Vehicle Model (9 DoF)_sfcn/3 -> __OutputSSForSFun__/3(__UniqueInportName__3__)
  Nonlinear Vehicle Model (9 DoF)_sfcn/4 -> __OutputSSForSFun__/4(__UniqueInportName__4__)
  Nonlinear Vehicle Model (9 DoF)_sfcn/5 -> __OutputSSForSFun__/5(__UniqueInportName__5__)
  Nonlinear Vehicle Model (9 DoF)_sfcn/6 -> __OutputSSForSFun__/6(__UniqueInportName__6__)
  Nonlinear Vehicle Model (9 DoF)_sfcn/7 -> __OutputSSForSFun__/7(__UniqueInportName__7__)
  Nonlinear Vehicle Model (9 DoF)_sfcn/8 -> __OutputSSForSFun__/8(__UniqueInportName__8__)
  Nonlinear Vehicle Model (9 DoF)_sfcn/9 -> __OutputSSForSFun__/9(__UniqueInportName__9__)
  Nonlinear Vehicle Model (9 DoF)_sfcn/10 -> __OutputSSForSFun__/10(__UniqueInportName__10__)
  __OutputSSForSFun__/1(long velocity [m/s]) -> long velocity [m/s]/1
  __OutputSSForSFun__/2(x-distance [m]) -> x-distance [m]/1
  __OutputSSForSFun__/3(y-distance [m]) -> y-distance [m]/1
  __OutputSSForSFun__/4(lat acceleration [m/s^2]) -> lat acceleration [m/s^2]/1
  __OutputSSForSFun__/5(lat velocity [m/s]) -> lat velocity [m/s]/1
  __OutputSSForSFun__/6(yaw rate [rad/s]) -> yaw rate [rad/s]/1
  __OutputSSForSFun__/7(wheel speed FL [rad/s]) -> wheel speed FL [rad/s]/1
  __OutputSSForSFun__/8(wheel speed FR [rad/s]) -> wheel speed FR [rad/s]/1
  __OutputSSForSFun__/9(wheel speed RL [rad/s]) -> wheel speed RL [rad/s]/1
  __OutputSSForSFun__/10(wheel speed RR [rad/s]) -> wheel speed RR [rad/s]/1

== system MPC_Extended_Plant_Simulink/Subsystem1/Regerence Generator ==
  note: yawr_ref
  note: nonlinear response
  note: delta
  note: u
  steering wheel angle [rad] : Inport
  long velocity [m/s] : Inport  Port=2
  MATLAB Function : MATLAB Function  TreatAsAtomicUnit=on
  MATLAB Function1 : MATLAB Function  TreatAsAtomicUnit=on
  Transfer Fcn : TransferFcn  Numerator=[par.wn^2*par.tau par.wn^2]  Denominator=[1 2*par.kseta*par.wn par.wn^2]
  steering ratio : Gain  Gain=1/ par.i_steer
  reference yaw rate [rad/s] : Outport  VectorParamsAs1DForOutWhenUnconnected=off
  wires:
  steering wheel angle [rad]/1 -> steering ratio/1
  steering ratio/1 -> MATLAB Function/1(delta)
  long velocity [m/s]/1 -> MATLAB Function1/2(u), MATLAB Function/2(u)
  MATLAB Function/1(yawr_ss) -> MATLAB Function1/1(yawr_ss)
  MATLAB Function1/1(yawr_sat) -> Transfer Fcn/1
  Transfer Fcn/1 -> reference yaw rate [rad/s]/1

== system MPC_Extended_Plant_Simulink/Subsystem1/Target Speed to Reach ==
  actual speed [m/s] : Inport
  " " : Lookup_n-D  NumberOfTableDimensions=1  BreakpointsForDimension1="[-10  0  10 30]"  IndexSearchMethod=Linear search  Table=[0.1 0.1 1 1]  ExtrapMethod=Clip  RemoveProtectionInput=on  UseLastTableValue=on  RndMeth=Simplest
  Add : Sum  Inputs=+-
  Add1 : Sum
  Gain : Gain  Gain=1000
  Gain1 : Gain  Gain=10
  Ground3 : Ground
  Integrator1 : Integrator  LimitOutput=on  UpperSaturationLimit=0.1  LowerSaturationLimit=-0.1
  Product : Product  RndMeth=Zero
  Product1 : Product  RndMeth=Zero
  Ramp6 : simulink/Sources/Ramp  slope=1  start=0  InitialOutput=0
  Saturation : Saturate  UpperLimit=1  LowerLimit=0
  Switch : Switch  Criteria=u2 > Threshold  Threshold=8  SaturateOnIntegerOverflow=off  InputSameDT=off
  low-pass (1 Hz) : TransferFcn  Denominator=[1/(2*pi) 1]
  "target pre-maneuver speed [m/s] " : Constant  Value=V_ref
  Drive torque [Nm] : Outport
  wires:
  actual speed [m/s]/1 -> low-pass (1 Hz)/1, Add/2
  "target pre-maneuver speed [m/s] "/1 -> Add/1
  Gain1/1 -> Integrator1/1
  Product/1 -> Add1/1
  Add/1 -> Product/1, Product1/1
  Product1/1 -> Gain1/1
  " "/1 -> Product1/2, Product/2
  low-pass (1 Hz)/1 -> " "/1
  Add1/1 -> Saturation/1
  Integrator1/1 -> Add1/2
  Ramp6/1 -> Switch/2
  Switch/1 -> Gain/1
  Ground3/1 -> Switch/1
  Saturation/1 -> Switch/3
  Gain/1 -> Drive torque [Nm]/1

== system MPC_Extended_Plant_Simulink/Subsystem1/steering system ==
  steering wheel angle [rad] : Inport
  Delay : TransportDelay  DelayTime=par.teta_ss
  Steering Dynamics : TransferFcn  Numerator=[par.wn_ss^2]  Denominator=[1 2*par.zeta_ss*par.wn_ss par.wn_ss^2]
  steering ratio : Gain  Gain=1/ par.i_steer
  wheel steer angle [rad] : Outport  VectorParamsAs1DForOutWhenUnconnected=off
  wires:
  steering wheel angle [rad]/1 -> steering ratio/1
  Delay/1 -> Steering Dynamics/1
  steering ratio/1 -> Delay/1
  Steering Dynamics/1 -> wheel steer angle [rad]/1

== system MPC_Extended_Plant_Simulink/Subsystem2/Driver Maneuver ==
  Constant1 : Constant
  Lookup Table1 : Lookup  InputValues=[0:0.1:3*pi/2 3*pi/2+eps]*0.7  Table=sin([0:0.1:3*pi/2 3*pi/2+eps])  LookUpMeth=Interpolation-Use End Values  SaturateOnIntegerOverflow=off
  Lookup Table2 : Lookup  InputValues=[3*pi/2:0.1:2*pi 2*pi+eps]*0.7  Table=sin([3*pi/2:0.1:2*pi 2*pi+eps])  LookUpMeth=Interpolation-Use End Values  SaturateOnIntegerOverflow=off
  Ramp2 : simulink/Sources/Ramp  slope=1  start=10  InitialOutput=0
  Ramp6 : simulink/Sources/Ramp  slope=pi  start=10  InitialOutput=0
  Ramp7 : simulink/Sources/Ramp  slope=pi  start=10+0.5  InitialOutput=0
  Sine Wave : Sin  TimeSource=Use external signal  Amplitude=30/180*pi  Frequency=2*pi*0.2  SampleTime=0
  Subtract1 : Sum  Inputs=+++
  Terminator1 : Terminator
  amplitude : Gain  Gain=120
  deg2rad : Gain  Gain=pi / 180
  steering wheel angle [rad] : Outport  VectorParamsAs1DForOutWhenUnconnected=off
  wires:
  Ramp6/1 -> Lookup Table1/1
  Ramp7/1 -> Lookup Table2/1
  Lookup Table2/1 -> Subtract1/2
  Lookup Table1/1 -> Subtract1/1
  Constant1/1 -> Subtract1/3
  Subtract1/1 -> amplitude/1
  amplitude/1 -> deg2rad/1
  Ramp2/1 -> Sine Wave/1
  deg2rad/1 -> steering wheel angle [rad]/1
  Sine Wave/1 -> Terminator1/1

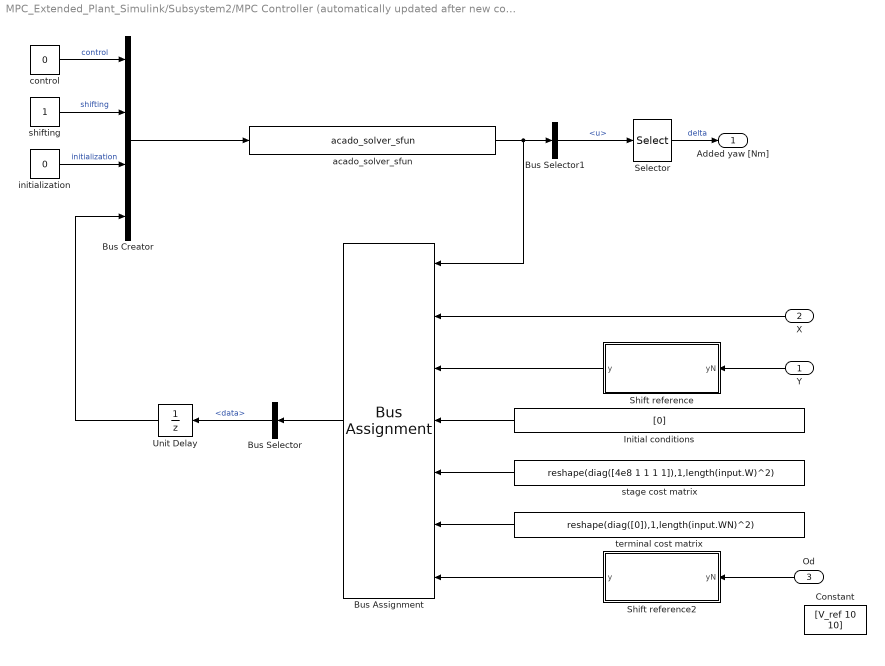
== system MPC_Extended_Plant_Simulink/Subsystem2/MPC Controller (automatically updated after new code generation) ==
  Y : Inport
  X : Inport  Port=2
  Od : Inport  Port=3
  Bus Assignment : BusAssignment  AssignedSignals=data.x0,data.y,data.yN,data.W,data.WN,data.od
  Bus Creator : BusCreator  Inputs=4  OutDataTypeStr=Bus: ACADOinput
  Bus Selector : BusSelector  OutputSignals=data
  Bus Selector1 : BusSelector  OutputSignals=data.u
  Constant : Constant  Value=[V_ref 10 10]
  Initial conditions : Constant  Value=[0]
  Selector : Selector  InputPortWidth=Np*4  IndexOptions=Starting index (dialog)  Indices=1  OutputSizes=4
  Shift reference : MATLAB Function  TreatAsAtomicUnit=on
  Shift reference2 : MATLAB Function  TreatAsAtomicUnit=on
  Unit Delay : UnitDelay  InitialCondition=init  SampleTime=Ts  HasFrameUpgradeWarning=on
  acado_solver_sfun : S-Function  FunctionName=acado_solver_sfun  SFunctionDeploymentMode=off  EnableBusSupport=off  mask(Legacy Function){SFunctionSpec=acado_step(ACADOinput u1[1], ACADOoutput y1[1]), ShowSpec=on}
      mask prompts: ShowSpec "Display function specification"
      mask help:
      | This block allows you to call the legacy functions specified by the following Legacy Code Tool definition:
      | def.SFunctionName = 'acado_solver_sfun';
      | def.OutputFcnSpec = 'acado_step(ACADOinput u1[1], ACADOoutput y1[1])';
      | def.StartFcnSpec = 'acado_initialize( void )';
      | def.TerminateFcnSpec = 'acado_cleanup( void )';
      | def.HeaderFiles = {'acado_common.h', 'acado_solver_sfunction.h'};
      | def.SourceFiles = {'acado_solver.c', 'acado_integrator.c', 'acado_auxiliary_functions.c', 'acado_solver_sfunction.c', 'acado_qpoases3_interface.c', 'qpoases3\src\Bounds.c', 'qpoases3\src\Constraints.c', 'qpoases3\src\Indexlist.c', 'qpoases3\src\Matrices.c', 'qpoases3\src\MessageHandling.c', 'qpoases3\src\Options.c', 'qpoases3\src\Flipper.c', 'qpoases3\src\QProblem.c', 'qpoases3\src\QProblemB.c', 'qpoases3\src\Utils.c'};
      mask Help: <p>This block was generated automatically by the Legacy Code Tool. For detailed help on this tool, call<a href="matlab:legacy_code('help')"> legacy_code('help')</a>.</p>
      mask Callback ShowSpec:
      | if strcmp(get_param(gcbh, 'ShowSpec'), 'on')
      |   set_param(gcbh, 'MaskDisplay', sprintf('fprintf(''%s'');', get_param(gcbh, 'SFunctionSpec')));
      | else
      |   set_param(gcbh, 'MaskDisplay', sprintf('fprintf(''%s'');', get_param(gcbh, 'FunctionName')));
      | end
      mask Display: fprintf('acado_step(ACADOinput u1[1], ACADOoutput y1[1])');
  control : Constant  Value=0  OutDataTypeStr=int32
  initialization : Constant  Value=0  OutDataTypeStr=int32
  shifting : Constant  OutDataTypeStr=int32
  stage cost matrix : Constant  Value=reshape(diag([4e8 1 1 1 1]),1,length(input.W)^2)
  terminal cost matrix : Constant  Value=reshape(diag([0]),1,length(input.WN)^2)
  Added yaw [Nm] : Outport
  wires:
  control/1 -> Bus Creator/1  "control"
  Bus Selector1/1 -> Selector/1  "<u>"
  initialization/1 -> Bus Creator/3  "initialization"
  acado_solver_sfun/1 -> Bus Selector1/1, Bus Assignment/1
  shifting/1 -> Bus Creator/2  "shifting"
  Bus Assignment/1 -> Bus Selector/1
  terminal cost matrix/1 -> Bus Assignment/6
  Initial conditions/1 -> Bus Assignment/4
  Shift reference/1(y) -> Bus Assignment/3
  stage cost matrix/1 -> Bus Assignment/5
  Bus Selector/1 -> Unit Delay/1  "<data>"
  Unit Delay/1 -> Bus Creator/4
  Bus Creator/1 -> acado_solver_sfun/1
  Selector/1 -> Added yaw [Nm]/1  "delta"
  Y/1 -> Shift reference/1(yN)
  X/1 -> Bus Assignment/2
  Shift reference2/1(y) -> Bus Assignment/7
  Od/1 -> Shift reference2/1(yN)
